simulink model "teste_ignore_simulink"  (R2018a)
settings: Solver=FixedStepAuto  StartTime=0.0  StopTime=tfinal  FixedStep=dt  RelTol=1e-3
values from neighbouring files (symbols this model uses):
  psi0 = 0*pi/180    (= 0)    [Trabalho_nSimples.m]
  yaw0 = 0    [Trabalho_nSimples.m]
settings Model: Creator=Adm  LastModifiedBy=Adm

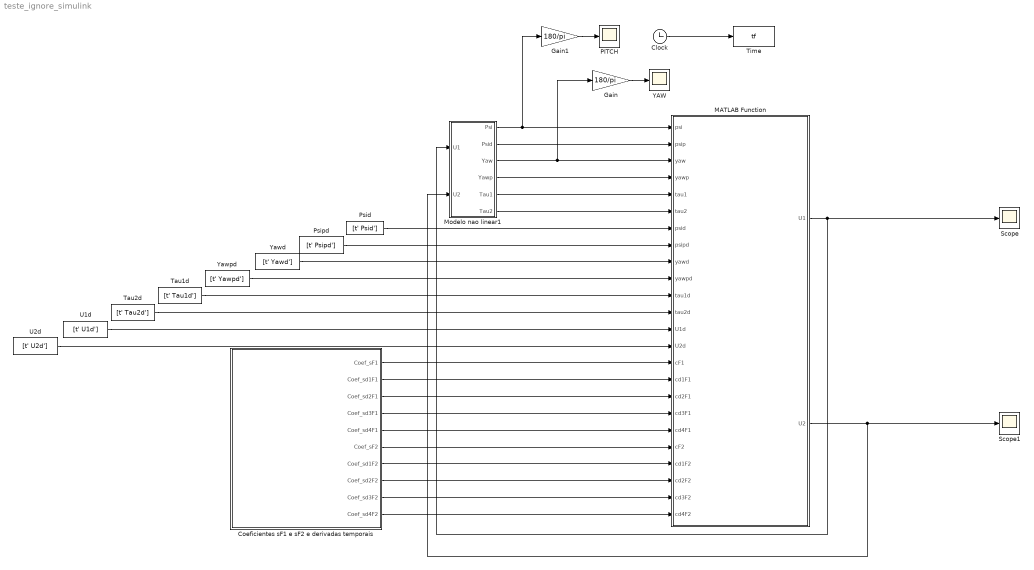
== system teste_ignore_simulink ==
  Clock : Clock
  Coeficientes sF1 e sF2 e derivadas temporais : Subsystem
  Gain : Gain  Gain=180/pi
  Gain1 : Gain  Gain=180/pi
  MATLAB Function : MATLAB Function  TreatAsAtomicUnit=on
  Modelo nao linear1 : Subsystem
  PITCH : Scope
  Psid : FromWorkspace  VariableName=[t' Psid']  OutDataTypeStr=double  SampleTime=0
  Psipd : FromWorkspace  VariableName=[t' Psipd']  OutDataTypeStr=double  SampleTime=0
  Scope : Scope
  Scope1 : Scope
  Tau1d : FromWorkspace  VariableName=[t' Tau1d']  OutDataTypeStr=double  SampleTime=0
  Tau2d : FromWorkspace  VariableName=[t' Tau2d']  OutDataTypeStr=double  SampleTime=0
  Time : ToWorkspace  VariableName=tf  SampleTime=-1
  U1d : FromWorkspace  VariableName=[t' U1d']  SampleTime=0  OutputAfterFinalValue=Holding final value
  U2d : FromWorkspace  VariableName=[t' U2d']  SampleTime=0  OutputAfterFinalValue=Holding final value
  YAW : Scope
  Yawd : FromWorkspace  VariableName=[t' Yawd']  OutDataTypeStr=double  SampleTime=0
  Yawpd : FromWorkspace  VariableName=[t' Yawpd']  OutDataTypeStr=double  SampleTime=0
  wires:
  MATLAB Function/1(U1) -> Modelo nao linear1/1(U1), Scope/1
  MATLAB Function/2(U2) -> Scope1/1, Modelo nao linear1/2(U2)
  Clock/1 -> Time/1
  Psipd/1 -> MATLAB Function/8(psipd)
  Tau1d/1 -> MATLAB Function/11(tau1d)
  Yawd/1 -> MATLAB Function/9(yawd)
  Psid/1 -> MATLAB Function/7(psid)
  Yawpd/1 -> MATLAB Function/10(yawpd)
  U1d/1 -> MATLAB Function/13(U1d)
  U2d/1 -> MATLAB Function/14(U2d)
  Tau2d/1 -> MATLAB Function/12(tau2d)
  Coeficientes sF1 e sF2 e derivadas temporais/10(Coef_sd4F2) -> MATLAB Function/24(cd4F2)
  Coeficientes sF1 e sF2 e derivadas temporais/9(Coef_sd3F2) -> MATLAB Function/23(cd3F2)
  Coeficientes sF1 e sF2 e derivadas temporais/8(Coef_sd2F2) -> MATLAB Function/22(cd2F2)
  Coeficientes sF1 e sF2 e derivadas temporais/7(Coef_sd1F2) -> MATLAB Function/21(cd1F2)
  Coeficientes sF1 e sF2 e derivadas temporais/6(Coef_sF2) -> MATLAB Function/20(cF2)
  Coeficientes sF1 e sF2 e derivadas temporais/5(Coef_sd4F1) -> MATLAB Function/19(cd4F1)
  Coeficientes sF1 e sF2 e derivadas temporais/4("Coef_sd3F1 ") -> MATLAB Function/18(cd3F1)
  Coeficientes sF1 e sF2 e derivadas temporais/3(Coef_sd2F1) -> MATLAB Function/17(cd2F1)
  Coeficientes sF1 e sF2 e derivadas temporais/2(Coef_sd1F1) -> MATLAB Function/16(cd1F1)
  Coeficientes sF1 e sF2 e derivadas temporais/1(Coef_sF1) -> MATLAB Function/15(cF1)
  Modelo nao linear1/2(Psid) -> MATLAB Function/2(psip)
  Modelo nao linear1/1(Psi) -> Gain1/1, MATLAB Function/1(psi)
  Modelo nao linear1/3(Yaw) -> Gain/1, MATLAB Function/3(yaw)
  Modelo nao linear1/4(Yawp) -> MATLAB Function/4(yawp)
  Modelo nao linear1/5(Tau1) -> MATLAB Function/5(tau1)
  Modelo nao linear1/6(Tau2) -> MATLAB Function/6(tau2)
  Gain/1 -> YAW/1
  Gain1/1 -> PITCH/1

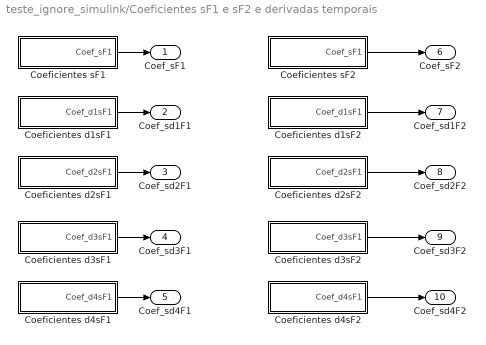
== system teste_ignore_simulink/Coeficientes sF1 e sF2 e derivadas temporais ==
  Coeficientes d1sF1 : Subsystem
  Coeficientes d1sF2 : Subsystem
  Coeficientes d2sF1 : Subsystem
  Coeficientes d2sF2 : Subsystem
  Coeficientes d3sF1 : Subsystem
  Coeficientes d3sF2 : Subsystem
  Coeficientes d4sF1 : Subsystem
  Coeficientes d4sF2 : Subsystem
  Coeficientes sF1 : Subsystem
  Coeficientes sF2 : Subsystem
  Coef_sF1 : Outport
  Coef_sd1F1 : Outport  Port=2
  Coef_sd2F1 : Outport  Port=3
  "Coef_sd3F1 " : Outport  Port=4
  Coef_sd4F1 : Outport  Port=5
  Coef_sF2 : Outport  Port=6
  Coef_sd1F2 : Outport  Port=7
  Coef_sd2F2 : Outport  Port=8
  Coef_sd3F2 : Outport  Port=9
  Coef_sd4F2 : Outport  Port=10
  wires:
  Coeficientes sF1/1(Coef_sF1) -> Coef_sF1/1
  Coeficientes d1sF1/1(Coef_d1sF1) -> Coef_sd1F1/1
  Coeficientes d2sF1/1(Coef_d2sF1) -> Coef_sd2F1/1
  Coeficientes sF2/1(Coef_sF1) -> Coef_sF2/1
  Coeficientes d1sF2/1(Coef_d1sF1) -> Coef_sd1F2/1
  Coeficientes d2sF2/1(Coef_d2sF1) -> Coef_sd2F2/1
  Coeficientes d3sF1/1(Coef_d3sF1) -> "Coef_sd3F1 "/1
  Coeficientes d4sF1/1(Coef_d4sF1) -> Coef_sd4F1/1
  Coeficientes d4sF2/1(Coef_d4sF1) -> Coef_sd4F2/1
  Coeficientes d3sF2/1(Coef_d3sF1) -> Coef_sd3F2/1

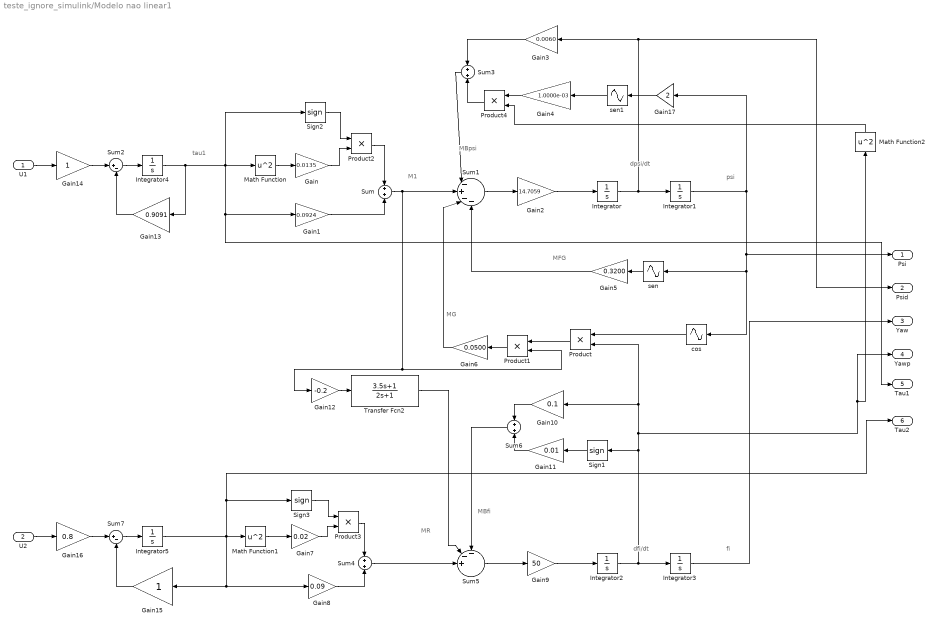
== system teste_ignore_simulink/Modelo nao linear1 ==
  note: MBfi
  note: MR
  note: psi
  note: MFG
  note: tau1
  note: M1
  note: MG
  note: MBpsi
  note: fi
  note: dfi/dt
  note: dpsi/dt
  U1 : Inport
  U2 : Inport  Port=2
  Gain : Gain  Gain=0.0135
  Gain1 : Gain  Gain=0.0924
  Gain10 : Gain  Gain=0.1
  Gain11 : Gain  Gain=0.01
  Gain12 : Gain  Gain=-0.2
  Gain13 : Gain  Gain=0.9091
  Gain14 : Gain
  Gain15 : Gain
  Gain16 : Gain  Gain=0.8
  Gain17 : Gain  Gain=2
  Gain2 : Gain  Gain=14.7059
  Gain3 : Gain  Gain=0.0060
  Gain4 : Gain  Gain=1.0000e-03
  Gain5 : Gain  Gain=0.3200
  Gain6 : Gain  Gain=0.0500
  Gain7 : Gain  Gain=0.02
  Gain8 : Gain  Gain=0.09
  Gain9 : Gain  Gain=50
  Integrator{,2,4..5} (4 alike) : Integrator
  Integrator1 : Integrator  InitialCondition=psi0
  Integrator3 : Integrator  InitialCondition=yaw0
  Math Function : Math  Operator=square  SaturateOnIntegerOverflow=on
  Math Function1 : Math  Operator=square  SaturateOnIntegerOverflow=on
  Math Function2 : Math  Operator=square  SaturateOnIntegerOverflow=on
  Product{,1..4} (5 alike) : Product
  Sign1 : Signum  ZeroCross=off
  Sign2 : Signum  ZeroCross=off
  Sign3 : Signum  ZeroCross=off
  Sum{,3..4,6} (4 alike) : Sum
  Sum1 : Sum  Inputs=|-+--
  Sum2 : Sum  Inputs=|+-
  Sum5 : Sum  Inputs=--+||
  Sum7 : Sum  Inputs=|+-
  Transfer Fcn2 : TransferFcn  Numerator=[3.5 1]  Denominator=[2 1]
  cos : Sin  TimeSource=Use external signal  Phase=pi/2  SampleTime=0
  sen : Sin  TimeSource=Use external signal  SampleTime=0
  sen1 : Sin  TimeSource=Use external signal  SampleTime=0
  Psi : Outport
  Psid : Outport  Port=2
  Yaw : Outport  Port=3
  Yawp : Outport  Port=4
  Tau1 : Outport  Port=5
  Tau2 : Outport  Port=6
  wires:
  Gain14/1 -> Sum2/1
  Integrator5/1 -> Math Function1/1, Sign3/1, Tau2/1, Gain8/1, Gain15/1
  Sum2/1 -> Integrator4/1
  Gain15/1 -> Sum7/2
  Gain13/1 -> Sum2/2
  U1/1 -> Gain14/1
  Gain16/1 -> Sum7/1
  Sum7/1 -> Integrator5/1
  Integrator4/1 -> Gain13/1, Sign2/1, Math Function/1, Tau1/1, Gain1/1
  Math Function/1 -> Gain/1
  Gain1/1 -> Sum/2
  Sum1/1 -> Gain2/1
  Gain2/1 -> Integrator/1
  Gain3/1 -> Sum3/1
  Sum3/1 -> Sum1/1
  Sum/1 -> Product1/2, Gain12/1, Sum1/2
  Integrator1/1 -> cos/1, sen/1, Psi/1, Gain17/1
  sen/1 -> Gain5/1
  Gain5/1 -> Sum1/4
  cos/1 -> Product/1
  Integrator2/1 -> Product/2, Gain10/1, Yawp/1, Math Function2/1, Sign1/1, Integrator3/1
  Product1/1 -> Gain6/1
  Gain6/1 -> Sum1/3
  Product/1 -> Product1/1
  Math Function1/1 -> Gain7/1
  Gain8/1 -> Sum4/2
  Sum5/1 -> Gain9/1
  Gain9/1 -> Integrator2/1
  Sign1/1 -> Gain11/1
  Gain10/1 -> Sum6/1
  Gain11/1 -> Sum6/2
  U2/1 -> Gain16/1
  Integrator3/1 -> Yaw/1
  Sum4/1 -> Sum5/3
  Sum6/1 -> Sum5/1
  Transfer Fcn2/1 -> Sum5/2
  Gain12/1 -> Transfer Fcn2/1
  Sign2/1 -> Product2/1
  Gain/1 -> Product2/2
  Product2/1 -> Sum/1
  Gain7/1 -> Product3/2
  Sign3/1 -> Product3/1
  Product3/1 -> Sum4/1
  sen1/1 -> Gain4/1
  Gain17/1 -> sen1/1
  Integrator/1 -> Psid/1, Gain3/1, Integrator1/1
  Gain4/1 -> Product4/1
  Product4/1 -> Sum3/2
  Math Function2/1 -> Product4/2

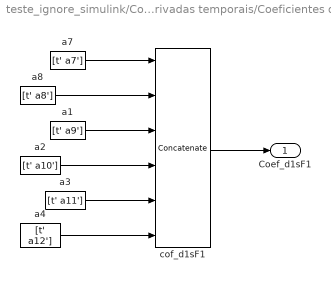
== system teste_ignore_simulink/Coeficientes sF1 e sF2 e derivadas temporais/Coeficientes d1sF1 ==
  a1 : FromWorkspace  VariableName=[t' a9']  SampleTime=0
  a2 : FromWorkspace  VariableName=[t' a10']  SampleTime=0
  a3 : FromWorkspace  VariableName=[t' a11']  SampleTime=0
  a4 : FromWorkspace  VariableName=[t' a12']  SampleTime=0
  a7 : FromWorkspace  VariableName=[t' a7']  SampleTime=0
  a8 : FromWorkspace  VariableName=[t' a8']  SampleTime=0
  cof_d1sF1 : Concatenate  NumInputs=6  ConcatenateDimension=2
  Coef_d1sF1 : Outport
  wires:
  cof_d1sF1/1 -> Coef_d1sF1/1
  a7/1 -> cof_d1sF1/1
  a8/1 -> cof_d1sF1/2
  a2/1 -> cof_d1sF1/4
  a1/1 -> cof_d1sF1/3
  a4/1 -> cof_d1sF1/6
  a3/1 -> cof_d1sF1/5

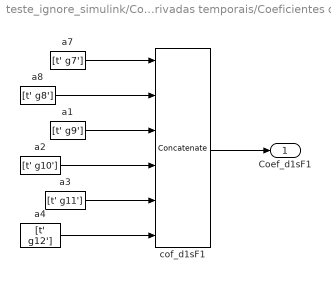
== system teste_ignore_simulink/Coeficientes sF1 e sF2 e derivadas temporais/Coeficientes d1sF2 ==
  a1 : FromWorkspace  VariableName=[t' g9']  SampleTime=0
  a2 : FromWorkspace  VariableName=[t' g10']  SampleTime=0
  a3 : FromWorkspace  VariableName=[t' g11']  SampleTime=0
  a4 : FromWorkspace  VariableName=[t' g12']  SampleTime=0
  a7 : FromWorkspace  VariableName=[t' g7']  SampleTime=0
  a8 : FromWorkspace  VariableName=[t' g8']  SampleTime=0
  cof_d1sF1 : Concatenate  NumInputs=6  ConcatenateDimension=2
  Coef_d1sF1 : Outport
  wires:
  cof_d1sF1/1 -> Coef_d1sF1/1
  a7/1 -> cof_d1sF1/1
  a8/1 -> cof_d1sF1/2
  a2/1 -> cof_d1sF1/4
  a1/1 -> cof_d1sF1/3
  a4/1 -> cof_d1sF1/6
  a3/1 -> cof_d1sF1/5

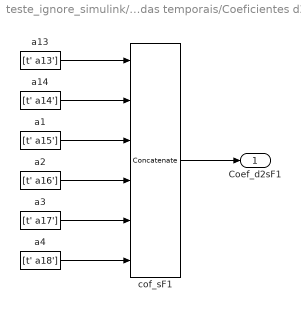
== system teste_ignore_simulink/Coeficientes sF1 e sF2 e derivadas temporais/Coeficientes d2sF1 ==
  a1 : FromWorkspace  VariableName=[t' a15']  SampleTime=0
  a13 : FromWorkspace  VariableName=[t' a13']  SampleTime=0
  a14 : FromWorkspace  VariableName=[t' a14']  SampleTime=0
  a2 : FromWorkspace  VariableName=[t' a16']  SampleTime=0
  a3 : FromWorkspace  VariableName=[t' a17']  SampleTime=0
  a4 : FromWorkspace  VariableName=[t' a18']  SampleTime=0
  cof_sF1 : Concatenate  NumInputs=6  ConcatenateDimension=2
  Coef_d2sF1 : Outport
  wires:
  cof_sF1/1 -> Coef_d2sF1/1
  a13/1 -> cof_sF1/1
  a14/1 -> cof_sF1/2
  a1/1 -> cof_sF1/3
  a2/1 -> cof_sF1/4
  a3/1 -> cof_sF1/5
  a4/1 -> cof_sF1/6

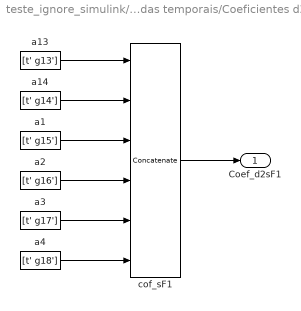
== system teste_ignore_simulink/Coeficientes sF1 e sF2 e derivadas temporais/Coeficientes d2sF2 ==
  a1 : FromWorkspace  VariableName=[t' g15']  SampleTime=0
  a13 : FromWorkspace  VariableName=[t' g13']  SampleTime=0
  a14 : FromWorkspace  VariableName=[t' g14']  SampleTime=0
  a2 : FromWorkspace  VariableName=[t' g16']  SampleTime=0
  a3 : FromWorkspace  VariableName=[t' g17']  SampleTime=0
  a4 : FromWorkspace  VariableName=[t' g18']  SampleTime=0
  cof_sF1 : Concatenate  NumInputs=6  ConcatenateDimension=2
  Coef_d2sF1 : Outport
  wires:
  cof_sF1/1 -> Coef_d2sF1/1
  a13/1 -> cof_sF1/1
  a14/1 -> cof_sF1/2
  a1/1 -> cof_sF1/3
  a2/1 -> cof_sF1/4
  a3/1 -> cof_sF1/5
  a4/1 -> cof_sF1/6

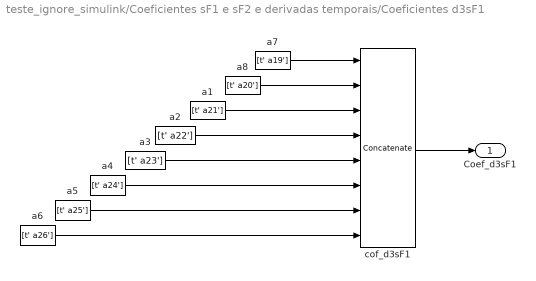
== system teste_ignore_simulink/Coeficientes sF1 e sF2 e derivadas temporais/Coeficientes d3sF1 ==
  a1 : FromWorkspace  VariableName=[t' a21']  SampleTime=0
  a2 : FromWorkspace  VariableName=[t' a22']  SampleTime=0
  a3 : FromWorkspace  VariableName=[t' a23']  SampleTime=0
  a4 : FromWorkspace  VariableName=[t' a24']  SampleTime=0
  a5 : FromWorkspace  VariableName=[t' a25']  SampleTime=0
  a6 : FromWorkspace  VariableName=[t' a26']  SampleTime=0
  a7 : FromWorkspace  VariableName=[t' a19']  SampleTime=0
  a8 : FromWorkspace  VariableName=[t' a20']  SampleTime=0
  cof_d3sF1 : Concatenate  NumInputs=8  ConcatenateDimension=2
  Coef_d3sF1 : Outport
  wires:
  cof_d3sF1/1 -> Coef_d3sF1/1
  a7/1 -> cof_d3sF1/1
  a8/1 -> cof_d3sF1/2
  a2/1 -> cof_d3sF1/4
  a1/1 -> cof_d3sF1/3
  a4/1 -> cof_d3sF1/6
  a3/1 -> cof_d3sF1/5
  a6/1 -> cof_d3sF1/8
  a5/1 -> cof_d3sF1/7

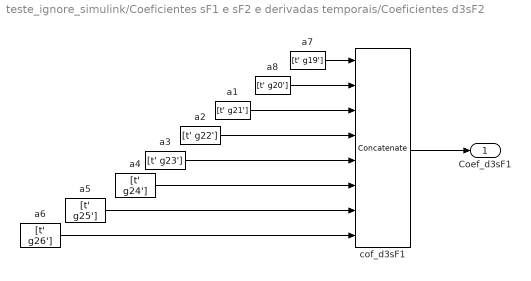
== system teste_ignore_simulink/Coeficientes sF1 e sF2 e derivadas temporais/Coeficientes d3sF2 ==
  a1 : FromWorkspace  VariableName=[t' g21']  SampleTime=0
  a2 : FromWorkspace  VariableName=[t' g22']  SampleTime=0
  a3 : FromWorkspace  VariableName=[t' g23']  SampleTime=0
  a4 : FromWorkspace  VariableName=[t' g24']  SampleTime=0
  a5 : FromWorkspace  VariableName=[t' g25']  SampleTime=0
  a6 : FromWorkspace  VariableName=[t' g26']  SampleTime=0
  a7 : FromWorkspace  VariableName=[t' g19']  SampleTime=0
  a8 : FromWorkspace  VariableName=[t' g20']  SampleTime=0
  cof_d3sF1 : Concatenate  NumInputs=8  ConcatenateDimension=2
  Coef_d3sF1 : Outport
  wires:
  cof_d3sF1/1 -> Coef_d3sF1/1
  a7/1 -> cof_d3sF1/1
  a8/1 -> cof_d3sF1/2
  a2/1 -> cof_d3sF1/4
  a1/1 -> cof_d3sF1/3
  a4/1 -> cof_d3sF1/6
  a3/1 -> cof_d3sF1/5
  a6/1 -> cof_d3sF1/8
  a5/1 -> cof_d3sF1/7

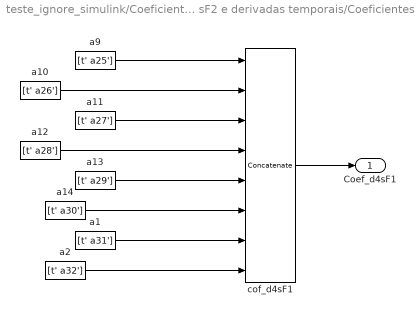
== system teste_ignore_simulink/Coeficientes sF1 e sF2 e derivadas temporais/Coeficientes d4sF1 ==
  a1 : FromWorkspace  VariableName=[t' a31']  SampleTime=0
  a10 : FromWorkspace  VariableName=[t' a26']  SampleTime=0
  a11 : FromWorkspace  VariableName=[t' a27']  SampleTime=0
  a12 : FromWorkspace  VariableName=[t' a28']  SampleTime=0
  a13 : FromWorkspace  VariableName=[t' a29']  SampleTime=0
  a14 : FromWorkspace  VariableName=[t' a30']  SampleTime=0
  a2 : FromWorkspace  VariableName=[t' a32']  SampleTime=0
  a9 : FromWorkspace  VariableName=[t' a25']  SampleTime=0
  cof_d4sF1 : Concatenate  NumInputs=8  ConcatenateDimension=2
  Coef_d4sF1 : Outport
  wires:
  cof_d4sF1/1 -> Coef_d4sF1/1
  a14/1 -> cof_d4sF1/6
  a9/1 -> cof_d4sF1/1
  a12/1 -> cof_d4sF1/4
  a13/1 -> cof_d4sF1/5
  a10/1 -> cof_d4sF1/2
  a11/1 -> cof_d4sF1/3
  a2/1 -> cof_d4sF1/8
  a1/1 -> cof_d4sF1/7

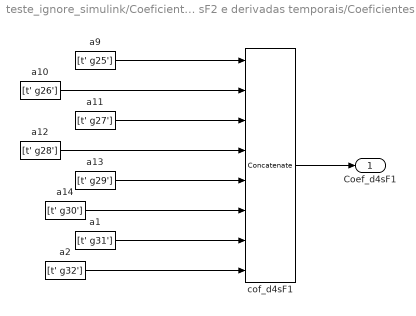
== system teste_ignore_simulink/Coeficientes sF1 e sF2 e derivadas temporais/Coeficientes d4sF2 ==
  a1 : FromWorkspace  VariableName=[t' g31']  SampleTime=0
  a10 : FromWorkspace  VariableName=[t' g26']  SampleTime=0
  a11 : FromWorkspace  VariableName=[t' g27']  SampleTime=0
  a12 : FromWorkspace  VariableName=[t' g28']  SampleTime=0
  a13 : FromWorkspace  VariableName=[t' g29']  SampleTime=0
  a14 : FromWorkspace  VariableName=[t' g30']  SampleTime=0
  a2 : FromWorkspace  VariableName=[t' g32']  SampleTime=0
  a9 : FromWorkspace  VariableName=[t' g25']  SampleTime=0
  cof_d4sF1 : Concatenate  NumInputs=8  ConcatenateDimension=2
  Coef_d4sF1 : Outport
  wires:
  cof_d4sF1/1 -> Coef_d4sF1/1
  a14/1 -> cof_d4sF1/6
  a9/1 -> cof_d4sF1/1
  a12/1 -> cof_d4sF1/4
  a13/1 -> cof_d4sF1/5
  a10/1 -> cof_d4sF1/2
  a11/1 -> cof_d4sF1/3
  a2/1 -> cof_d4sF1/8
  a1/1 -> cof_d4sF1/7

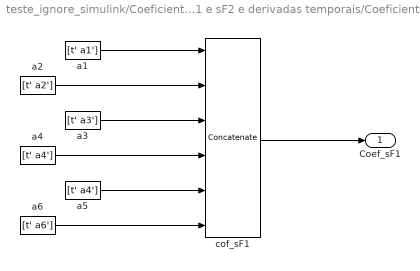
== system teste_ignore_simulink/Coeficientes sF1 e sF2 e derivadas temporais/Coeficientes sF1 ==
  a1 : FromWorkspace  VariableName=[t' a1']  SampleTime=0
  a2 : FromWorkspace  VariableName=[t' a2']  SampleTime=0
  a3 : FromWorkspace  VariableName=[t' a3']  SampleTime=0
  a4 : FromWorkspace  VariableName=[t' a4']  SampleTime=0
  a5 : FromWorkspace  VariableName=[t' a4']  SampleTime=0
  a6 : FromWorkspace  VariableName=[t' a6']  SampleTime=0
  cof_sF1 : Concatenate  NumInputs=6  ConcatenateDimension=2
  Coef_sF1 : Outport
  wires:
  cof_sF1/1 -> Coef_sF1/1
  a4/1 -> cof_sF1/4
  a3/1 -> cof_sF1/3
  a2/1 -> cof_sF1/2
  a1/1 -> cof_sF1/1
  a5/1 -> cof_sF1/5
  a6/1 -> cof_sF1/6

== system teste_ignore_simulink/Coeficientes sF1 e sF2 e derivadas temporais/Coeficientes sF2 ==
  a1 : FromWorkspace  VariableName=[t' g1']  SampleTime=0
  a2 : FromWorkspace  VariableName=[t' g2']  SampleTime=0
  a3 : FromWorkspace  VariableName=[t' g3']  SampleTime=0
  a4 : FromWorkspace  VariableName=[t' g4']  SampleTime=0
  a5 : FromWorkspace  VariableName=[t' g4']  SampleTime=0
  a6 : FromWorkspace  VariableName=[t' g6']  SampleTime=0
  cof_sF1 : Concatenate  NumInputs=6  ConcatenateDimension=2
  Coef_sF1 : Outport
  wires:
  cof_sF1/1 -> Coef_sF1/1
  a4/1 -> cof_sF1/4
  a3/1 -> cof_sF1/3
  a2/1 -> cof_sF1/2
  a1/1 -> cof_sF1/1
  a5/1 -> cof_sF1/5
  a6/1 -> cof_sF1/6

== matlab function teste_ignore_simulink/MATLAB Function ==
  data: psi input; U1 output; U2 output; psip input; yaw input; yawp input; tau1 input; tau2 input; psid input; psipd input; yawd input; yawpd input; tau1d input; tau2d input; U1d input; U2d input; cF1 input; cd1F1 input; cd2F1 input; cd3F1 input; cd4F1 input; cF2 input; cd1F2 input; cd2F2 input; cd3F2 input; cd4F2 input
function [U1,U2] = fcn(psi, psip, yaw, yawp, tau1, tau2, psid, psipd, yawd, yawpd, tau1d, tau2d, U1d, U2d, cF1, cd1F1, cd2F1,cd3F1, cd4F1, cF2, cd1F2, cd2F2,cd3F2, cd4F2)
K01=1;K11=1;K02=1;K12=1;K21=1;K22=1;
limU1_sup=20;limU2_sup=20;limU1_inf=-20;limU2_inf=-20;
% Inicialização
    cF1 = cF1'; cd1F1 = cd1F1'; cd2F1 = cd2F1'; cd3F1 = cd3F1';
    cF2 = cF2'; cd1F2 = cd1F2'; cd2F2 = cd2F2'; cd3F2 = cd3F2';
%     disp(cd2F1)
%     disp(size(cd2F1));
%     porta3 = 0;porta4 = 0;porta5 = 0;porta6 = 0;
%     porta7 = 0;porta8 = 0;
  % Etapa 01 - Variáveis Incrementais (Erro de Trajetória)
    sPsi = psi - psid; sPsip = psip - psipd; sYaw= yaw - yawd; sYawp = yawp - yawpd;
    sTau1 = tau1 - tau1d; sTau2 = tau2 - tau2d;
%   % Etapa 02 - Construção da Saída Plana e suas Derivadas Temporais
    sF1   =   cF1*[sPsi; sPsip; sYaw; sYawp;sTau1;sTau2];
    d1sF1 = cd1F1*[sPsi; sPsip; sYaw; sYawp;sTau1;sTau2];%     disp(d1sF1)
    d2sF1 = cd2F1*[sPsi; sPsip; sYaw; sYawp;sTau1;sTau2];
    
    sF2   =   cF1*[sPsi; sPsip; sYaw; sYawp;sTau1;sTau2];
    d1sF2 = cd1F2*[sPsi; sPsip; sYaw; sYawp;sTau1;sTau2];
    d2sF2 = cd2F2*[sPsi; sPsip; sYaw; sYawp;sTau1;sTau2];
  % Etapa 03 - Termos de Correção em Malha Fechada
    tC1 = - K21*d2sF1 - K11*d1sF1 - K01*sF1; 
    tC2 = - K22*d2sF2 - K12*d1sF2 - K02*sF2;
%     
%   % Etapa 04 - Gerando a Expressão Final para os Controladores
%     
%     % Calculando os Coeficientes de sU1 e sU2

      M  = [  cF1(1,1) cF1(1,2) cF1(1,3) cF1(1,4) cF1(1,5) cF1(1,6) 0 0; 
              cd1F1(1,1) cd1F1(1,2) cd1F1(1,3) cd1F1(1,4) cd1F1(1,5) cd1F1(1,6) 0 0;
              cd2F1(1,1) cd2F1(1,2) cd2F1(1,3) cd2F1(1,4) cd2F1(1,5) cd2F1(1,6) 0 0;
              cd3F1(1,1) cd3F1(1,2) cd3F1(1,3) cd3F1(1,4) cd3F1(1,5) cd3F1(1,6) cd3F1(1,7) cd3F1(1,8);
              
              cF2(1,1) cF2(1,2) cF2(1,3) cF2(1,4) cF2(1,5) cF2(1,6) 0 0; 
              cd1F2(1,1) cd1F2(1,2) cd1F2(1,3) cd1F2(1,4) cd1F2(1,5) cd1F2(1,6) 0 0;
              cd2F2(1,1) cd2F2(1,2) cd2F2(1,3) cd2F2(1,4) cd2F2(1,5) cd2F2(1,6) 0 0;
              cd3F2(1,1) cd3F2(1,2) cd3F2(1,3) cd3F2(1,4) cd3F2(1,5) cd3F2(1,6) cd3F2(1,7) cd3F2(1,8);];
      
       iM = M^(-1);
      cU1 = iM(4,:);
      cU2 = iM(8,:);
    
    % Expressão dos Sinais de Controle Incrementais
      sU1 = cU1*[sF1; d1sF1; d2sF2; tC1; sF2; d1sF2; d2sF2;  tC2];
      sU2 = cU2*[sF1; d1sF1; d2sF2; tC1; sF2; d1sF2; d2sF2;  tC2];
  
    % Expressão Final do Sinais de Controle "U1" e "U2"
      temp_U1 = sU1 + U1d;
      temp_U2 = sU2 + U2d;
      
    % Saturação dos Atuadores
      U1 = min(limU1_sup, max(limU1_inf, temp_U1));
      U2 = min(limU2_sup, max(limU2_inf, temp_U2));
      U1 = 0;
      U2 = 0;











end
